simulink model "p11"  (R2021b)
settings: Solver=VariableStepAuto  StartTime=0.0  StopTime=10.0  MaxStep=0.001  RelTol=1e-3
libraries: simulink x1
settings Model: Creator=user  LastModifiedBy=user

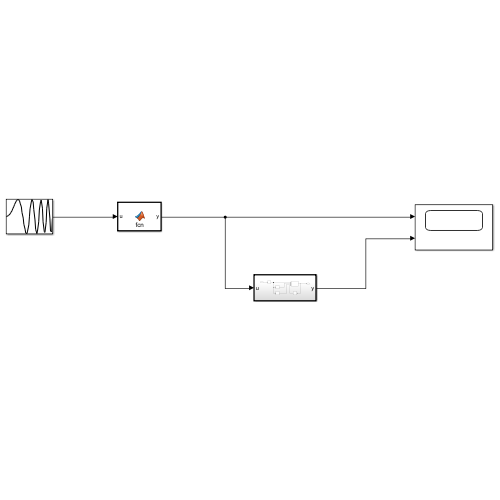
[thumbnail: Simulink's stored preview of the top-level diagram]
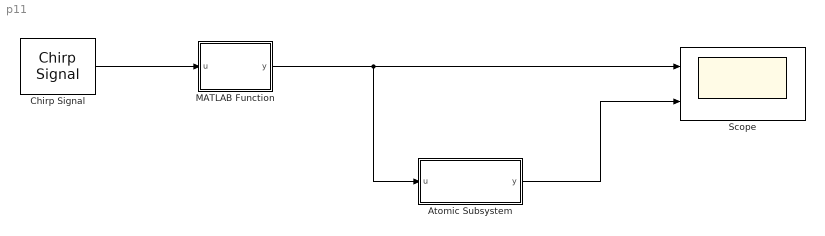
== system p11 ==
  Atomic Subsystem : Subsystem  TreatAsAtomicUnit=on
  Chirp Signal : simulink/Sources/Chirp Signal  f1=1/2/pi  T=1e1  f2=1000/2/pi
  MATLAB Function : MATLAB Function  TreatAsAtomicUnit=on
  Scope : Scope  NumInputPorts=2
  wires:
  Chirp Signal/1 -> MATLAB Function/1(u)
  MATLAB Function/1(y) -> Scope/1, Atomic Subsystem/1(u)
  Atomic Subsystem/1(y) -> Scope/2

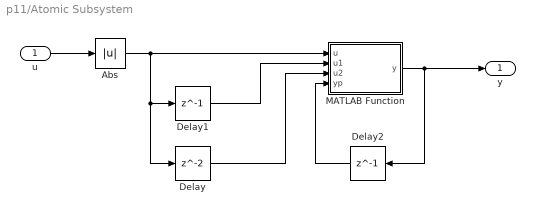
== system p11/Atomic Subsystem ==
  u : Inport
  Abs : Abs
  Delay : Delay
  Delay1 : Delay  DelayLength=1
  Delay2 : Delay  DelayLength=1  InitialCondition=1
  MATLAB Function : MATLAB Function  TreatAsAtomicUnit=on
  y : Outport
  wires:
  u/1 -> Abs/1
  Abs/1 -> Delay/1, Delay1/1, MATLAB Function/1(u)
  Delay1/1 -> MATLAB Function/2(u1)
  Delay/1 -> MATLAB Function/3(u2)
  Delay2/1 -> MATLAB Function/4(yp)
  MATLAB Function/1(y) -> y/1, Delay2/1

== matlab function p11/MATLAB Function ==
  data: u input; y output
function y = fcn(u)

T = linspace(0,10,10000);
syms t 
h = piecewise( (0<=t)<=1,1 ,t<0,0 ,t>1,0);

p = eval(subs(h,t,T));

[num,den] = impulse2tf(p,T);

sys = tf(num,den);

y = sys.;

== matlab function p11/Atomic Subsystem/MATLAB Function ==
  data: u input; y output; u1 input; u2 input; yp input
function y = fcn(u,u1,u2,yp)

    if((u1>u2)&&(u1>u))
            y = u;

    else
        y =yp;
    end
